simulink model "Parent"  (R2023a)
settings: Solver=FixedStepDiscrete  StartTime=0.0  StopTime=inf  RelTol=1e-3
undefined symbols (not defined in the file): Data_Display, Data_Display1, Data_Display2, Data_Display3, Data_Display4, Data_Display5, Parent_1
libraries: androidcommunicationlib x9, androiduilib x6, androidaudiovideolib x1, androidsensorlib x1
settings Model: Creator=darsh  LastModifiedBy=agarw_crynhxp
settings OptimizationCC: EnhancedBackFolding=on  PassReuseOutputArgsAs=Individual arguments  ZeroExternalMemoryAtStartup=off  ZeroInternalMemoryAtStartup=off  MaxStackSize=64  OptimizeBlockOrder=speed  DifferentSizesBufferReuse=on  OptimizationCustomize=off  EfficientTunableParamExpr=on
settings DebuggingCC: ParameterTunabilityLossMsg=error
settings HardwareCC: ProdBitPerPointer=32  ProdBitPerSizeT=32  ProdBitPerPtrDiffT=32  ProdLargestAtomicInteger=Long  ProdLargestAtomicFloat=Double  ProdWordSize=32  ProdHWDeviceType=ARM Compatible->ARM Cortex  UseEmbeddedCoderFeatures=off  UseSimulinkCoderFeatures=off
settings SFSimCC: MATLABDynamicMemAlloc=off
settings RTWCC: Description=Embedded Coder  SystemTargetFile=ert.tlc  HardwareBoard=Android Device  TLCOptions="-aInlineSetEventsForThisBaseRateFcn=TLC_FALSE -aSuppressMultiTaskScheduler=TLC_FALSE  -aRateBasedStepFcn=0"  TemplateMakefile=ert_default_tmf  RTWVerbose=off  Toolchain=Android SDK/NDK Tools
settings CodeAppCC: ForceParamTrailComments=on  IgnoreCustomStorageClasses=off  OperatorAnnotations=on  SimulinkDataObjDesc=on  SFDataObjDesc=on  InsertBlockDesc=on
settings ERTTargetCC: SupportNonInlinedSFcns=on

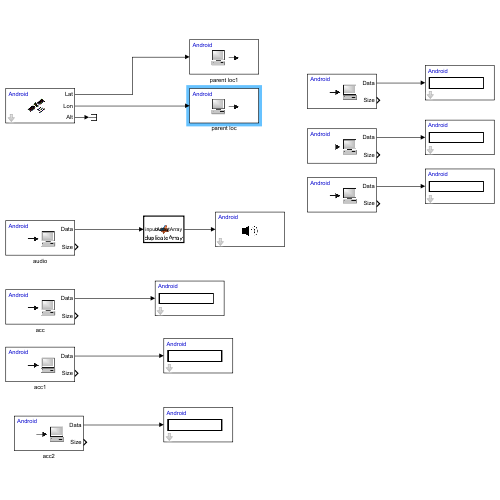
[thumbnail: Simulink's stored preview of the top-level diagram]
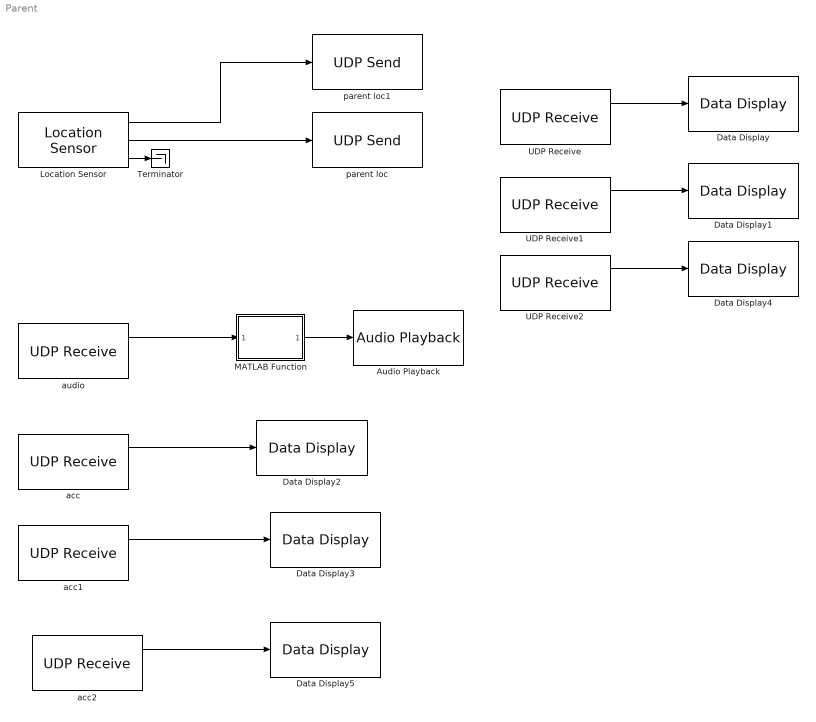
== system Parent ==
  Audio Playback : androidaudiovideolib/Audio Playback  SampleFreq=44100  AudioSamplingFreq=44100  SampleTime=0.1  DeviceStr=0  QueueDuration=0  BlockPlatform=Android
  Data Display : androiduilib/Data Display  DataDisplayId=Parent_1/Data_Display  Format=Float  Precision=6  SimulateUsing=Code generation  blockPlatform=Android
  Data Display1 : androiduilib/Data Display  DataDisplayId=Parent_1/Data_Display1  Format=Float  Precision=6  SimulateUsing=Code generation  blockPlatform=Android
  Data Display2 : androiduilib/Data Display  DataDisplayId=Parent_1/Data_Display2  Format=Float  Precision=6  SimulateUsing=Code generation  blockPlatform=Android
  Data Display3 : androiduilib/Data Display  DataDisplayId=Parent_1/Data_Display3  Format=Float  Precision=6  SimulateUsing=Code generation  blockPlatform=Android
  Data Display4 : androiduilib/Data Display  DataDisplayId=Parent_1/Data_Display4  Format=Float  Precision=6  SimulateUsing=Code generation  blockPlatform=Android
  Data Display5 : androiduilib/Data Display  DataDisplayId=Parent_1/Data_Display5  Format=Float  Precision=6  SimulateUsing=Code generation  blockPlatform=Android
  Location Sensor : androidsensorlib/Location Sensor  OutputVector=off  SampleTime=0.1  BlockPlatform=Android
  MATLAB Function : MATLAB Function  TreatAsAtomicUnit=on
  Terminator : Terminator
  UDP Receive : androidcommunicationlib/UDP Receive  localURL='0.0.0.0'  localPort=50000  remoteURL='0.0.0.0'  remotePort=-1  recvBufferSize=8192  signalDatatype=uint8  dims=255  isVarSize=off  showBlockingTime=off  blockingTime=0  sampletime=0.01  blockPlatform=Android
  UDP Receive1 : androidcommunicationlib/UDP Receive  localURL='0.0.0.0'  localPort=55000  remoteURL='0.0.0.0'  remotePort=-1  recvBufferSize=8192  signalDatatype=uint8  dims=255  isVarSize=off  showBlockingTime=off  blockingTime=0  sampletime=0.01  blockPlatform=Android
  UDP Receive2 : androidcommunicationlib/UDP Receive  localURL='0.0.0.0'  localPort=60000  remoteURL='0.0.0.0'  remotePort=-1  recvBufferSize=8192  signalDatatype=uint8  dims=255  isVarSize=off  showBlockingTime=off  blockingTime=0  sampletime=0.01  blockPlatform=Android
  acc : androidcommunicationlib/UDP Receive  localURL='0.0.0.0'  localPort=20000  remoteURL='0.0.0.0'  remotePort=-1  recvBufferSize=8192  signalDatatype=uint8  dims=255  isVarSize=off  showBlockingTime=off  blockingTime=0  sampletime=0.01  blockPlatform=Android
  acc1 : androidcommunicationlib/UDP Receive  localURL='0.0.0.0'  localPort=15000  remoteURL='0.0.0.0'  remotePort=-1  recvBufferSize=8192  signalDatatype=uint8  dims=255  isVarSize=off  showBlockingTime=off  blockingTime=0  sampletime=0.01  blockPlatform=Android
  acc2 : androidcommunicationlib/UDP Receive  localURL='0.0.0.0'  localPort=25000  remoteURL='0.0.0.0'  remotePort=-1  recvBufferSize=8192  signalDatatype=uint8  dims=255  isVarSize=off  showBlockingTime=off  blockingTime=0  sampletime=0.01  blockPlatform=Android
  audio : androidcommunicationlib/UDP Receive  localURL='0.0.0.0'  localPort=30000  remoteURL='0.0.0.0'  remotePort=-1  recvBufferSize=8192  signalDatatype=int16  dims=441  isVarSize=off  showBlockingTime=off  blockingTime=0  sampletime=0.01  blockPlatform=Android
  parent loc : androidcommunicationlib/UDP Send  remoteURL='10.7.27.78'  remotePort=45000  localURL='0.0.0.0'  localPortSource=Automatically determine  localPort=-1  sampletime=-1  blockPlatform=Android  separateLengthPort=0
  parent loc1 : androidcommunicationlib/UDP Send  remoteURL='10.7.27.78'  remotePort=40000  localURL='0.0.0.0'  localPortSource=Automatically determine  localPort=-1  sampletime=-1  blockPlatform=Android  separateLengthPort=0
  wires:
  Location Sensor/3 -> Terminator/1
  Location Sensor/1 -> parent loc1/1
  audio/1 -> MATLAB Function/1(inputArray)
  MATLAB Function/1(outputArray) -> Audio Playback/1
  Location Sensor/2 -> parent loc/1
  UDP Receive/1 -> Data Display/1
  UDP Receive1/1 -> Data Display1/1
  UDP Receive2/1 -> Data Display4/1
  acc/1 -> Data Display2/1
  acc1/1 -> Data Display3/1
  acc2/1 -> Data Display5/1

== matlab function Parent/MATLAB Function ==
  data: inputArray input; outputArray output
function outputArray = duplicateArray(inputArray)
    % Check if the inputArray is a column vector (nx1)
    if size(inputArray, 2) ~= 1
        error('Input array must be an nx1 column vector.');
    end

    % Duplicate the inputArray horizontally to create an nx2 array
    outputArray = [inputArray, inputArray];
end
